simulink model "LongiAcc"  (R2019a)
settings: Solver=VariableStepAuto  StartTime=0.0  StopTime=10.0  RelTol=1e-3
values from neighbouring files (symbols this model uses):
  cl = 50000    [LongAccParams.m]
  I = 1.5    [LongAccParams.m]
  m = 250    [LongAccParams.m]
  R = 0.32    [LongAccParams.m]
settings Model: Creator=a33shahi  LastModifiedBy=a33shahi

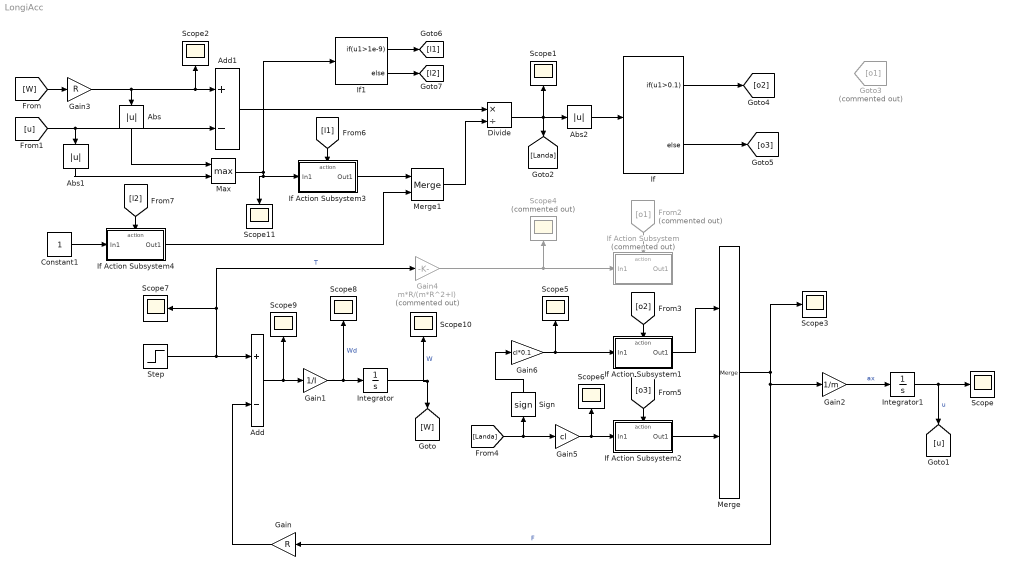
== system LongiAcc ==
  Abs : Abs
  Abs1 : Abs
  Abs2 : Abs
  Add : Sum  Inputs=+-
  Add1 : Sum  Inputs=+-
  Constant1 : Constant
  Divide : Product  Inputs=*/
  From2 : From  Commented=on  GotoTag=o1
  Gain : Gain  Gain=R
  Gain1 : Gain  Gain=1/I
  Gain2 : Gain  Gain=1/m
  Gain3 : Gain  Gain=R
  Gain4 : Gain  Commented=on  Gain=m*R/(m*R^2+I)
  Gain5 : Gain  Gain=cl
  Gain6 : Gain  Gain=cl*0.1
  Goto3 : Goto  Commented=on  GotoTag=o1
  If : If  IfExpression=u1>0.1
  If Action Subsystem : Subsystem  Commented=on  TreatAsAtomicUnit=on
  If Action Subsystem1 : Subsystem  TreatAsAtomicUnit=on
  If Action Subsystem2 : Subsystem  TreatAsAtomicUnit=on
  If Action Subsystem3 : Subsystem  TreatAsAtomicUnit=on
  If Action Subsystem4 : Subsystem  TreatAsAtomicUnit=on
  If1 : If  IfExpression=u1>1e-9
  Integrator : Integrator  InitialCondition=0.0
  Integrator1 : Integrator
  Max : MinMax  Function=max  Inputs=2
  Merge : Merge
  Merge1 : Merge
  Scope{,1..3,5..11} (11 alike) : Scope
  Scope4 : Scope  Commented=on
  Sign : Signum
  Step : Step  Time=0  After=100  SampleTime=0
  wires:
  Step/1 -> Scope7/1, Gain4/1, Add/1  "T"
  Gain/1 -> Add/2
  Add/1 -> Scope9/1, Gain1/1
  Merge/1 -> Scope3/1, Gain/1, Gain2/1  "F"
  Gain1/1 -> Scope8/1, Integrator/1  "Wd"
  Integrator/1 -> Scope10/1, [W]  "W"
  Gain2/1 -> Integrator1/1  "ax"
  Integrator1/1 -> [u], Scope/1  "u"
  [W] -> Gain3/1
  Add1/1 -> Divide/1
  Divide/1 -> Abs2/1, Scope1/1, [Landa]
  If/1 -> [o2]
  If/2 -> [o3]
  From2/1 -> If Action Subsystem/Action
  Gain4/1 -> Scope4/1, If Action Subsystem/1(In1)
  [o2] -> If Action Subsystem1/Action
  Gain6/1 -> If Action Subsystem1/1(In1), Scope5/1
  If Action Subsystem1/1(Out1) -> Merge/1
  If Action Subsystem2/1(Out1) -> Merge/2
  [Landa] -> Sign/1, Gain5/1
  Gain5/1 -> Scope6/1, If Action Subsystem2/1(In1)
  [o3] -> If Action Subsystem2/Action
  Max/1 -> Scope11/1, If Action Subsystem3/1(In1), If1/1
  Merge1/1 -> Divide/2
  If Action Subsystem3/1(Out1) -> Merge1/1
  Constant1/1 -> If Action Subsystem4/1(In1)
  If Action Subsystem4/1(Out1) -> Merge1/2
  [l1] -> If Action Subsystem3/Action
  [l2] -> If Action Subsystem4/Action
  If1/1 -> [l1]
  If1/2 -> [l2]
  Gain3/1 -> Scope2/1, Add1/1, Abs/1
  [u] -> Abs1/1, Add1/2
  Abs2/1 -> If/1
  Abs/1 -> Max/1
  Abs1/1 -> Max/2
  Sign/1 -> Gain6/1

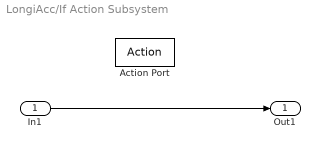
== system LongiAcc/If Action Subsystem ==
  In1 : Inport
  Action Port : ActionPort  ActionPortLabel=if(u1==0)
  Out1 : Outport
  wires:
  In1/1 -> Out1/1

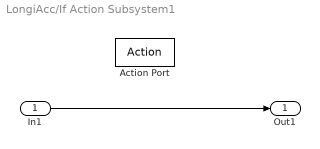
== system LongiAcc/If Action Subsystem1 ==
  In1 : Inport
  Action Port : ActionPort  ActionPortLabel=if(u1>0.1)
  Out1 : Outport
  wires:
  In1/1 -> Out1/1

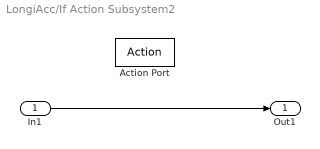
== system LongiAcc/If Action Subsystem2 ==
  In1 : Inport
  Action Port : ActionPort  ActionPortLabel=else
  Out1 : Outport
  wires:
  In1/1 -> Out1/1

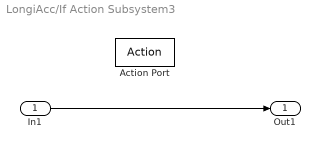
== system LongiAcc/If Action Subsystem3 ==
  In1 : Inport
  Action Port : ActionPort  ActionPortLabel=if(u1>1e-9)
  Out1 : Outport
  wires:
  In1/1 -> Out1/1

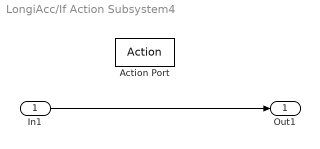
== system LongiAcc/If Action Subsystem4 ==
  In1 : Inport
  Action Port : ActionPort  ActionPortLabel=else
  Out1 : Outport
  wires:
  In1/1 -> Out1/1
